simulink model "SolveDiffEqn"  (R2023b)
settings: Solver=VariableStepAuto  StartTime=0.0  StopTime=10.0  RelTol=1e-3
settings Model: Creator=kasaoka  LastModifiedBy=kasaoka

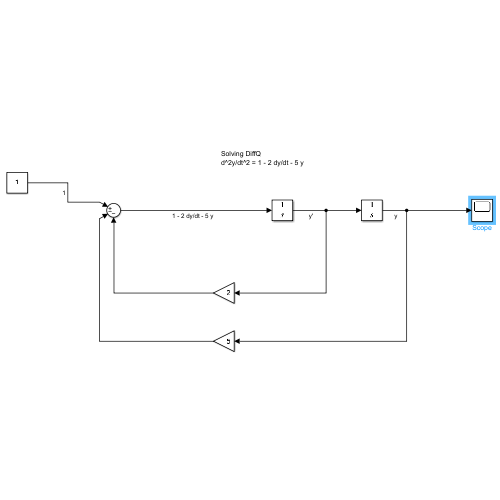
[thumbnail: Simulink's stored preview of the top-level diagram]
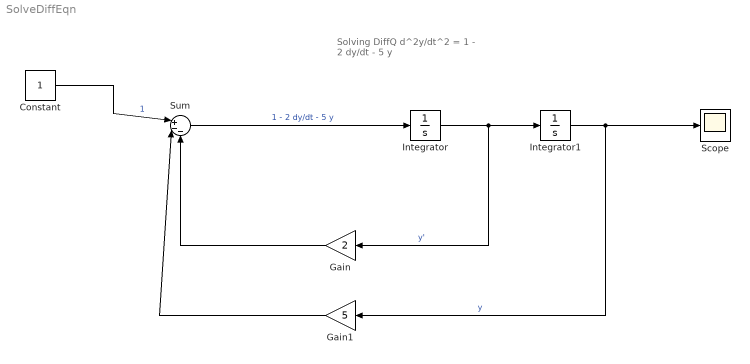
== system SolveDiffEqn ==
  note: Solving DiffQ
      | d^2y/dt^2 = 1 - 2 dy/dt - 5 y
  Constant : Constant
  Gain : Gain  Gain=2
  Gain1 : Gain  Gain=5
  Integrator : Integrator
  Integrator1 : Integrator
  Scope : Scope
  Sum : Sum  Inputs=|+--
  wires:
  Constant/1 -> Sum/1  "1"
  Sum/1 -> Integrator/1  "1 - 2 dy/dt - 5 y"
  Integrator1/1 -> Gain1/1, Scope/1  "y"
  Integrator/1 -> Gain/1, Integrator1/1  "y'"
  Gain/1 -> Sum/3
  Gain1/1 -> Sum/2
